simulink model "exercise_2_4"  (R2024b)
settings: Solver=VariableStepAuto  StartTime=0.0  StopTime=30  RelTol=1e-3
InitFcn:
  | disp('Loading EMG data...');
  | data = load('ES2_emg.mat');
  | 
  | signals = data.ES2_emg.signals; %30001x4
  | 
  | % Create time vector
  | Ts = 0.001;
  | 
  | num_samples = size(signals, 1);
  | 
  | time_vector = (0:num_samples-1)' * Ts;
  | 
  | raw_signals = [time_vector, signals];     % [Time, Data] 30001x5
  | 
  | disp('Data loaded and time vector created.');
  | 
  | 
  | %% FILTER DESIGN
  | 
  | Fs = 1/Ts;     % 1000 Hz
  | 
  | disp('Designing filters ...');
  | 
  | % NOTCH FILTER (50 Hz)
  | f0 = 50;
  | Q = 40;        % quality factor: higher means narrower notch
  | BW = f0 / Q;
  | d_notch = designfilt('bandstopiir', ...
  |     'FilterOrder', 2, ...
  |     'HalfPowerFrequency1', f0 - BW/2, ...
  |     'HalfPowerFrequency2', f0 + BW/2, ...
  |     'DesignMethod', 'butter', ...
  |     'SampleRate', Fs);
  | [b_notch, a_notch] = tf(d_notch);
  | 
  | % BANDPASS FILTER (30–450 Hz)
  | d_band = designfilt('bandpassiir', ...
  |     'FilterOrder', 4, ...
  |     'HalfPowerFrequency1', 30, ...
  |     'HalfPowerFrequency2', 450, ...
  |     'DesignMethod', 'butter', ...
  |     'SampleRate', Fs);
  | [b_band, a_band] = tf(d_band);
  | 
  | % LOWPASS FILTER (0.8 Hz)
  | d_low = designfilt('lowpassiir', ...
  |     'FilterOrder', 4, ...
  |     'HalfPowerFrequency', 0.8, ...
  |     'DesignMethod', 'butter', ...
  |     'SampleRate', Fs);
  | [b_low, a_low] = tf(d_low);
  | 
  | % LOWPASS AFTER DIVISION
  | f_cutoff = 0.5;
  | d_lowpass = designfilt('lowpassiir', ...
  |     'FilterOrder', 2, ...
  |     'HalfPowerFrequency', f_cutoff, ...
  |     'DesignMethod', 'butter', ...
  |     'SampleRate', Fs);
  | [b_low2, a_low2] = tf(d_lowpass);
  | 
  | disp('Filter coefficients generated');
undefined symbols (not defined in the file or in its folder): a_band, a_low, a_low2, a_notch, b_band, b_low, b_low2, b_notch, dspblkCoreblockFVToolHelper, gcbh
libraries: simulink x3, simulink_extras x1, vrlib x1
settings Model: Creator=Lenovo  LastModifiedBy=philg
settings RTWCC: GPUComputeCapability=3.5

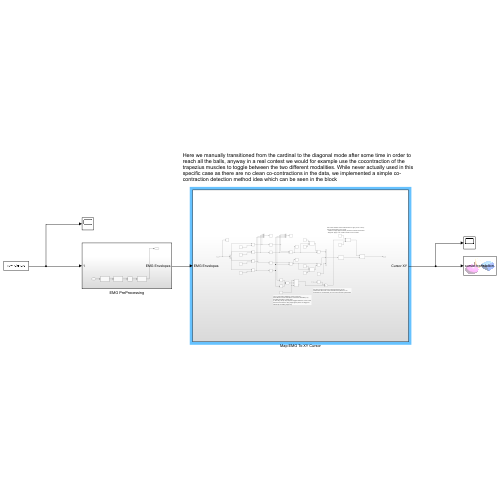
[thumbnail: Simulink's stored preview of the top-level diagram]
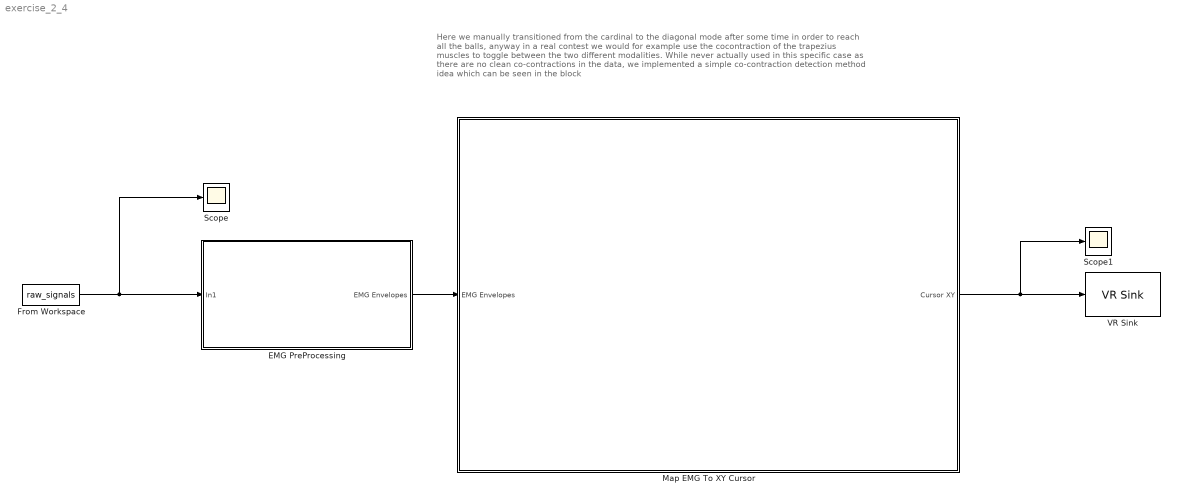
== system exercise_2_4 ==
  note: Here we manually transitioned from the cardinal to the diagonal mode after some time in order to reach all the balls, anyway in a real contest we would for example use the cocontraction of the trapezius muscles to toggle between the two different modalities. While never actually used in this specific case as there are no clean co-contractions in the data, we implemented a simple co-contraction detection method idea which can be seen in the block
  EMG PreProcessing : Subsystem
  From Workspace : FromWorkspace  VariableName=raw_signals  SampleTime=0.001  Interpolate=off  ZeroCross=off  OutputAfterFinalValue=Holding final value
  Map EMG To XY Cursor : Subsystem
  Scope : Scope
  Scope1 : Scope
  VR Sink : vrlib/VR Sink  InstantiateOnLoad=on  SampleTime=0.1  ViewEnable=on  RemoteChange=off  RemoteView=off  FieldsWritten=cursor.translation.3.1.1.double  WorldFileName=8_palline_color.wrl  AutoView=off  VideoDimensions=[]  AllowVariableSize=off  FigureProperties="{'Position', 'Name', 'Viewpoint', 'CameraBound', 'CameraDirection', 'CameraPosition', 'CameraUpVector', 'ZoomFactor', 'Antialiasing', 'Headlight', 'Lighting', 'Sound', 'StatusBar', 'Stereo3D', 'Stereo3DCameraOffset', 'Stereo3DHIT', 'ToolBar', 'Textures', 'Transparency', 'Triad', 'Wireframe', 'NavZones', 'NavMode', 'NavSpeed', 'CaptureFileFormat', 'CaptureFileName', 'Record2DCompressMethod', 'Record2DCompressQuality', 'Record2D', 'Record2DFileName', 'Record2DFPS', 'NavPanel'; [1.0000000000000000e+00   7.1666666666666515e+01   1.7066666666666665e+03   8.9600000000000000e+02], '', '_untitled_1', 'on', [0.0000000000000000e+00   0.0000000000000000e+00  -1.0000000000000000e+00], [0.0000000000000000e+00   0.0000000000000000e+00   0.0000000000000000e+00], [0.0000000000000000e+00   1.0000000000000000e+00   0.0000000000000000e+00], [1.0000000000000000e+00], 'on', 'on', 'on', 'on', 'on', 'off', [1.0000000149011612e-01], [0.0000000000000000e+00], 'on', 'on', 'on', 'none', 'off', 'off', 'fly', 'normal', 'tif', '%f_anim_%n.tif', 'auto', [7.5000000000000000e+01], 'off', '%f_anim_%n.avi', 'auto', 'halfbar'}"
  wires:
  From Workspace/1 -> EMG PreProcessing/1(In1), Scope/1
  EMG PreProcessing/1(EMG Envelopes) -> Map EMG To XY Cursor/1(EMG Envelopes)
  Map EMG To XY Cursor/1(Cursor XY) -> VR Sink/1, Scope1/1

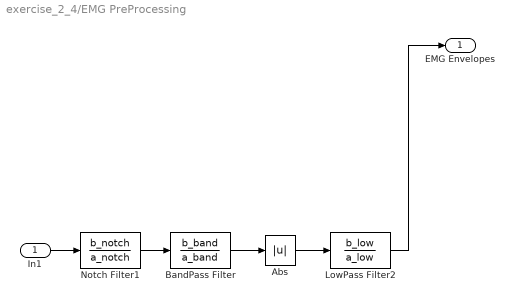
== system exercise_2_4/EMG PreProcessing ==
  In1 : Inport
  Abs : Abs  SaturateOnIntegerOverflow=off
  BandPass Filter : DiscreteFilter  LoadFcn=dspblkCoreblockFVToolHelper(gcbh,'load');  Numerator=b_band  Denominator=a_band
      settings: CopyFcn=dspblkCoreblockFVToolHelper(gcbh,'copy');  DeleteFcn=dspblkCoreblockFVToolHelper(gcbh,'close');  ModelCloseFcn=dspblkCoreblockFVToolHelper(gcbh,'close');  PreSaveFcn=dspblkCoreblockFVToolHelper(gcbh,'presave');  PostSaveFcn=dspblkCoreblockFVToolHelper(gcbh,'postsave');  CloseFcn=dspblkCoreblockFVToolHelper(gcbh,'close');
  LowPass Filter2 : DiscreteFilter  Numerator=b_low  Denominator=a_low
  Notch Filter1 : DiscreteFilter  LoadFcn=dspblkCoreblockFVToolHelper(gcbh,'load');  Numerator=b_notch  Denominator=a_notch
      settings: CopyFcn=dspblkCoreblockFVToolHelper(gcbh,'copy');  DeleteFcn=dspblkCoreblockFVToolHelper(gcbh,'close');  ModelCloseFcn=dspblkCoreblockFVToolHelper(gcbh,'close');  PreSaveFcn=dspblkCoreblockFVToolHelper(gcbh,'presave');  PostSaveFcn=dspblkCoreblockFVToolHelper(gcbh,'postsave');  CloseFcn=dspblkCoreblockFVToolHelper(gcbh,'close');
  EMG Envelopes : Outport
  wires:
  Abs/1 -> LowPass Filter2/1
  In1/1 -> Notch Filter1/1
  Notch Filter1/1 -> BandPass Filter/1
  BandPass Filter/1 -> Abs/1
  LowPass Filter2/1 -> EMG Envelopes/1

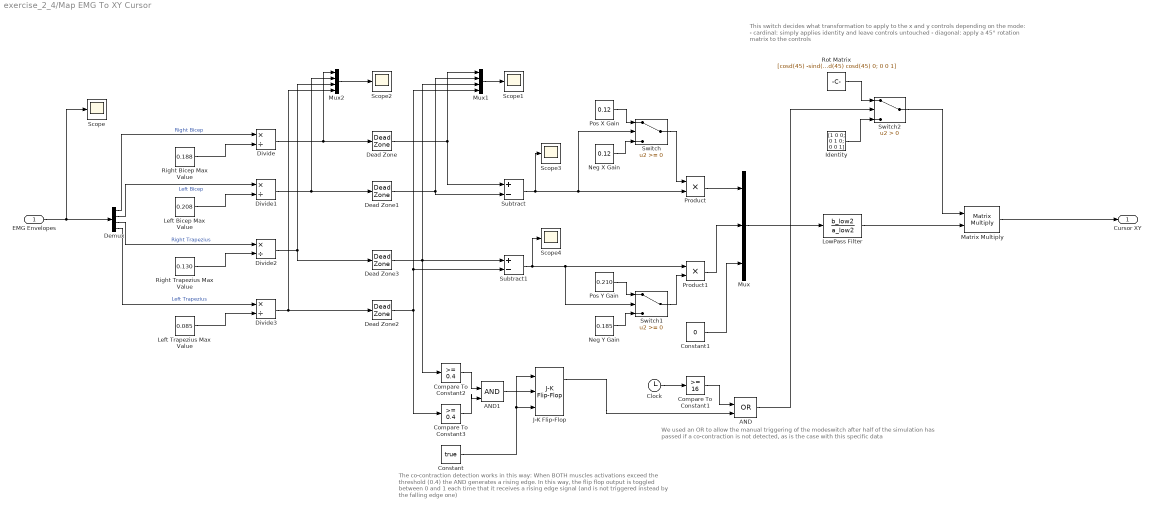
== system exercise_2_4/Map EMG To XY Cursor ==
  note: This switch decides what transformation to apply to the x and y controls depending on the mode:
      | - cardinal: simply applies identity and leave controls untouched
      | - diagonal: apply a 45° rotation matrix to the controls
  note: The co-contraction detection works in this way:
      | When BOTH muscles activations exceed the threshold (0.4)
      | the AND generates a rising edge.
      | In this way, the flip flop output is toggled between 0 and 1 each time that it receives a rising edge signal (and is not triggered instead by the falling edge one)
  note: We used an OR to allow the manual triggering of the modeswitch after half of the simulation has passed if a co-contraction is not detected, as is the case with this specific data
  EMG Envelopes : Inport
  AND : Logic  Operator=OR  IconShape=distinctive  AllPortsSameDT=off  OutDataTypeStr=boolean
  AND1 : Logic  IconShape=distinctive  AllPortsSameDT=off  OutDataTypeStr=boolean
  Clock : Clock
  Compare To Constant1 : simulink/Logic and Bit Operations/Compare To Constant  relop=>=  const=16  OutDataTypeStr=boolean
  Compare To Constant2 : simulink/Logic and Bit Operations/Compare To Constant  relop=>=  const=0.4  OutDataTypeStr=boolean
  Compare To Constant3 : simulink/Logic and Bit Operations/Compare To Constant  relop=>=  const=0.4  OutDataTypeStr=boolean
  Constant : Constant  Value=true
  Constant1 : Constant  Value=0
  Dead Zone : DeadZone  LowerValue=0  UpperValue=0.1
  Dead Zone1 : DeadZone  LowerValue=0  UpperValue=0.1
  Dead Zone2 : DeadZone  LowerValue=0  UpperValue=0.3
  Dead Zone3 : DeadZone  LowerValue=0  UpperValue=0.4
  Demux : Demux
  Divide{,1..3} (4 alike) : Product  Inputs=*/
  Identity : Constant  Value=[1 0 0; 0 1 0; 0 0 1]
  J-K Flip-Flop : simulink_extras/Flip Flops/J-K Flip-Flop  initial_condition=0
  Left Bicep Max Value : Constant  Value=0.208
  Left Trapezius Max Value : Constant  Value=0.085
  LowPass Filter : DiscreteFilter  LoadFcn=dspblkCoreblockFVToolHelper(gcbh,'load');  Numerator=b_low2  Denominator=a_low2
      settings: CopyFcn=dspblkCoreblockFVToolHelper(gcbh,'copy');  DeleteFcn=dspblkCoreblockFVToolHelper(gcbh,'close');  ModelCloseFcn=dspblkCoreblockFVToolHelper(gcbh,'close');  PreSaveFcn=dspblkCoreblockFVToolHelper(gcbh,'presave');  PostSaveFcn=dspblkCoreblockFVToolHelper(gcbh,'postsave');  CloseFcn=dspblkCoreblockFVToolHelper(gcbh,'close');
  Matrix Multiply : Product  Multiplication=Matrix(*)
  Mux : Mux  Inputs=3
  Mux1 : Mux
  Mux2 : Mux
  Neg X Gain : Constant  Value=0.12
  Neg Y Gain : Constant  Value=0.185
  Pos X Gain : Constant  Value=0.12
  Pos Y Gain : Constant  Value=0.210
  Product : Product
  Product1 : Product
  Right Bicep Max Value : Constant  Value=0.188
  Right Trapezius Max Value : Constant  Value=0.130
  Rot Matrix : Constant  Value=[cosd(45) -sind(45) 0; sind(45) cosd(45) 0; 0 0 1]
  Scope{,1..4} (5 alike) : Scope
  Subtract : Sum  Inputs=+-
  Subtract1 : Sum  Inputs=+-
  Switch : Switch  SaturateOnIntegerOverflow=off  InputSameDT=off
  Switch1 : Switch  SaturateOnIntegerOverflow=off  InputSameDT=off
  Switch2 : Switch  Criteria=u2 > Threshold  SaturateOnIntegerOverflow=off  InputSameDT=off
  Cursor XY : Outport
  wires:
  Constant1/1 -> Mux/3
  Demux/3 -> Divide2/1  "Right Trapezius"
  Demux/2 -> Divide1/1  "Left Bicep"
  Demux/4 -> Divide3/1  "Left Trapezius"
  Demux/1 -> Divide/1  "Right Bicep"
  EMG Envelopes/1 -> Scope/1, Demux/1
  Mux/1 -> LowPass Filter/1
  Mux1/1 -> Scope1/1
  Right Bicep Max Value/1 -> Divide/2
  Left Bicep Max Value/1 -> Divide1/2
  Right Trapezius Max Value/1 -> Divide2/2
  Left Trapezius Max Value/1 -> Divide3/2
  Divide/1 -> Mux2/1, Dead Zone/1
  Divide1/1 -> Mux2/2, Dead Zone1/1
  Divide2/1 -> Mux2/3, Dead Zone3/1
  Divide3/1 -> Mux2/4, Dead Zone2/1
  Mux2/1 -> Scope2/1
  Dead Zone/1 -> Mux1/1, Subtract/1
  Dead Zone1/1 -> Mux1/2, Subtract/2
  Subtract/1 -> Scope3/1, Switch/2, Product/2
  Subtract1/1 -> Switch1/2, Product1/1, Scope4/1
  Dead Zone3/1 -> Compare To Constant2/1, Subtract1/1, Mux1/3
  Dead Zone2/1 -> Compare To Constant3/1, Mux1/4, Subtract1/2
  Product/1 -> Mux/1
  Switch/1 -> Product/1
  Switch1/1 -> Product1/2
  Product1/1 -> Mux/2
  LowPass Filter/1 -> Matrix Multiply/2
  Matrix Multiply/1 -> Cursor XY/1
  Switch2/1 -> Matrix Multiply/1
  Rot Matrix/1 -> Switch2/1
  Identity/1 -> Switch2/3
  Clock/1 -> Compare To Constant1/1
  AND/1 -> Switch2/2
  Compare To Constant1/1 -> AND/1
  J-K Flip-Flop/1 -> AND/2
  Compare To Constant2/1 -> AND1/1
  Compare To Constant3/1 -> AND1/2
  AND1/1 -> J-K Flip-Flop/2
  Constant/1 -> J-K Flip-Flop/3, J-K Flip-Flop/1
  Neg X Gain/1 -> Switch/3
  Pos X Gain/1 -> Switch/1
  Neg Y Gain/1 -> Switch1/3
  Pos Y Gain/1 -> Switch1/1
